simulink model "gm_model_biquad_wfa_interface"  (R2020b)
settings: Solver=FixedStepAuto  StartTime=0.0  StopTime=1  RelTol=1e-3  EnableMultiTasking=on
undefined symbols (not defined in the file or in its folder): AXI4, Lite
libraries: axiinterfacelib x2
settings Model: Creator=pablo  LastModifiedBy=pablo
settings SolverCC: ConcurrentTasks=on  PositivePriorityOrder=on
settings OptimizationCC: EnhancedBackFolding=on  PassReuseOutputArgsAs=Individual arguments  ZeroExternalMemoryAtStartup=off  ZeroInternalMemoryAtStartup=off  MaxStackSize=64  OptimizeBlockOrder=speed  DifferentSizesBufferReuse=on  OptimizationCustomize=off  EfficientTunableParamExpr=on
settings DebuggingCC: ParameterTunabilityLossMsg=error
settings HardwareCC: ProdBitPerPointer=32  ProdBitPerSizeT=32  ProdBitPerPtrDiffT=32  ProdLargestAtomicInteger=Long  ProdLargestAtomicFloat=Double  ProdWordSize=32  ProdLongLongMode=on  ProdHWDeviceType=ARM Compatible->ARM Cortex  TargetBitPerPointer=64  TargetBitPerSizeT=64  TargetBitPerPtrDiffT=64  TargetLargestAtomicFloat=Float  TargetIntDivRoundTo=Zero  TargetEndianess=LittleEndian  TargetWordSize=64  TargetHWDeviceType=Intel->x86-64 (Windows64)
settings SFSimCC: MATLABDynamicMemAlloc=off
settings RTWCC: Description=Embedded Coder  SystemTargetFile=ert.tlc  HardwareBoard=Xilinx Zynq-7000 based board  TLCOptions="-aInlineSetEventsForThisBaseRateFcn=TLC_FALSE -aSuppressMultiTaskScheduler=TLC_FALSE  -aRateBasedStepFcn=0"  TemplateMakefile=ert_default_tmf  Toolchain=Linaro AArch32 Linux v6.3.1
settings CodeAppCC: ForceParamTrailComments=on  IgnoreCustomStorageClasses=off  OperatorAnnotations=on  SimulinkDataObjDesc=on  SFDataObjDesc=on  InsertBlockDesc=on

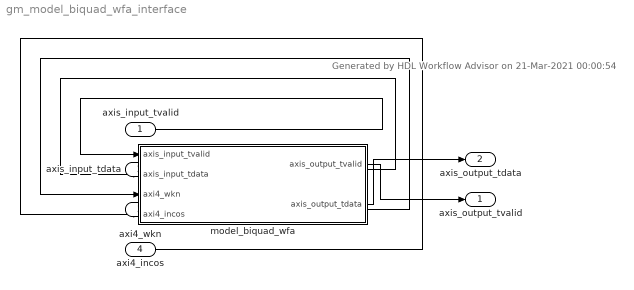
== system gm_model_biquad_wfa_interface ==
  note: Generated by HDL Workflow Advisor on 21-Mar-2021 00:00:54
  axis_input_tvalid : Inport
  axis_input_tdata : Inport  Port=2
  axi4_wkn : Inport  Port=3
  axi4_incos : Inport  Port=4
  model_biquad_wfa : Subsystem  TreatAsAtomicUnit=on  mask(AXI4-Lite/AXI4 Interface){}
      mask help:
      | This is an automatically generated subsystem block.
      | This contains the AXI interface blocks that communicate with the axis_goertzel_ip IPCore generated from model_biquad_wfa subsystem.
      mask Display: disp(sprintf('Xilinx Zynq \nAXI Interface'));
  axis_output_tvalid : Outport
  axis_output_tdata : Outport  Port=2
  wires:
  axis_input_tvalid/1 -> model_biquad_wfa/1(axis_input_tvalid)
  axis_input_tdata/1 -> model_biquad_wfa/2(axis_input_tdata)
  axi4_wkn/1 -> model_biquad_wfa/3(axi4_wkn)
  axi4_incos/1 -> model_biquad_wfa/4(axi4_incos)
  model_biquad_wfa/1(axis_output_tvalid) -> axis_output_tvalid/1
  model_biquad_wfa/2(axis_output_tdata) -> axis_output_tdata/1

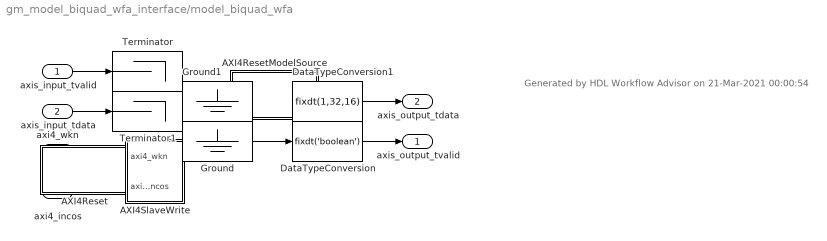
== system gm_model_biquad_wfa_interface/model_biquad_wfa ==
  note: Generated by HDL Workflow Advisor on 21-Mar-2021 00:00:54
  axis_input_tvalid : Inport
  axis_input_tdata : Inport  Port=2
  axi4_wkn : Inport  Port=3
  axi4_incos : Inport  Port=4
  AXI4Reset : Subsystem  mask(System Start){ShowInLibBrowser=0}
      mask prompts: ShowInLibBrowser "Simulink:masks:CustCodeMaskParam1_MP"
      settings: CopyFcn=cccopyfcn(gcb)  OpenFcn=ccopenfcn('System Start Function')
      mask Help: eval('feval(''rtwprivate'',''rtwhelpview'',''rtw_sys_start_block'')');
      mask Display: disp('System\nStart');
  AXI4ResetModelSource : Subsystem  mask(Model Source){ShowInLibBrowser=0}
      mask prompts: ShowInLibBrowser "Simulink:masks:CustCodeMaskParam1_MP"
      settings: CopyFcn=cccopyfcn(gcb)  OpenFcn=ccopenfcn('Model Source')
      mask Help: eval('feval(''rtwprivate'',''rtwhelpview'',''rtw_model_source_block'')');
      mask Display: disp('Model\nSource');
  AXI4SlaveWrite : Subsystem  Priority=1
  DataTypeConversion : DataTypeConversion  OutDataTypeStr=fixdt('boolean')  ConvertRealWorld=Stored Integer (SI)
  DataTypeConversion1 : DataTypeConversion  OutDataTypeStr=fixdt(1,32,16)  ConvertRealWorld=Stored Integer (SI)
  Ground : Ground
  Ground1 : Ground
  Terminator : Terminator
  Terminator1 : Terminator
  axis_output_tvalid : Outport
  axis_output_tdata : Outport  Port=2
  wires:
  axi4_wkn/1 -> AXI4SlaveWrite/1(axi4_wkn)
  axi4_incos/1 -> AXI4SlaveWrite/2(axi4_incos)
  axis_input_tvalid/1 -> Terminator/1
  axis_input_tdata/1 -> Terminator1/1
  DataTypeConversion/1 -> axis_output_tvalid/1
  Ground/1 -> DataTypeConversion/1
  DataTypeConversion1/1 -> axis_output_tdata/1
  Ground1/1 -> DataTypeConversion1/1

== system gm_model_biquad_wfa_interface/model_biquad_wfa/AXI4Reset ==

== system gm_model_biquad_wfa_interface/model_biquad_wfa/AXI4ResetModelSource ==

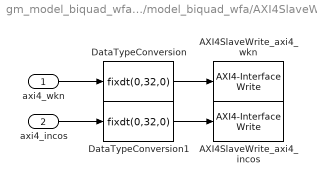
== system gm_model_biquad_wfa_interface/model_biquad_wfa/AXI4SlaveWrite ==
  axi4_wkn : Inport
  axi4_incos : Inport  Port=2
  AXI4SlaveWrite_axi4_incos : axiinterfacelib/AXI4-Interface Write  Priority=2  AXIInterfaceType=AXI4-Lite  DeviceName=/dev/mwipcore  RegisterOffset=hex2dec('100')  blockPlatform=ZYNQ  SimulateUsing=Interpreted execution
      settings: SourceProductBaseCode=ECZYNQ7000
  AXI4SlaveWrite_axi4_wkn : axiinterfacelib/AXI4-Interface Write  Priority=1  AXIInterfaceType=AXI4-Lite  DeviceName=/dev/mwipcore  RegisterOffset=hex2dec('104')  blockPlatform=ZYNQ  SimulateUsing=Interpreted execution
      settings: SourceProductBaseCode=ECZYNQ7000
  DataTypeConversion : DataTypeConversion  OutDataTypeStr=fixdt(0,32,0)  ConvertRealWorld=Stored Integer (SI)
  DataTypeConversion1 : DataTypeConversion  OutDataTypeStr=fixdt(0,32,0)  ConvertRealWorld=Stored Integer (SI)
  wires:
  DataTypeConversion/1 -> AXI4SlaveWrite_axi4_wkn/1
  axi4_incos/1 -> DataTypeConversion1/1
  axi4_wkn/1 -> DataTypeConversion/1
  DataTypeConversion1/1 -> AXI4SlaveWrite_axi4_incos/1
